simulink model "quad_copter_hybrid_vrft"  (R2016a)
settings: Solver=VariableStepAuto  StartTime=0.0  StopTime=10  RelTol=1e-3
undefined symbols (not defined in the file): DiscIntNeverNeededParam, HybridVRFTController, Mixer, PitchRateModel_dt, Ri_dt, Ts
settings Model: Creator=tibo  LastModifiedBy=tibo

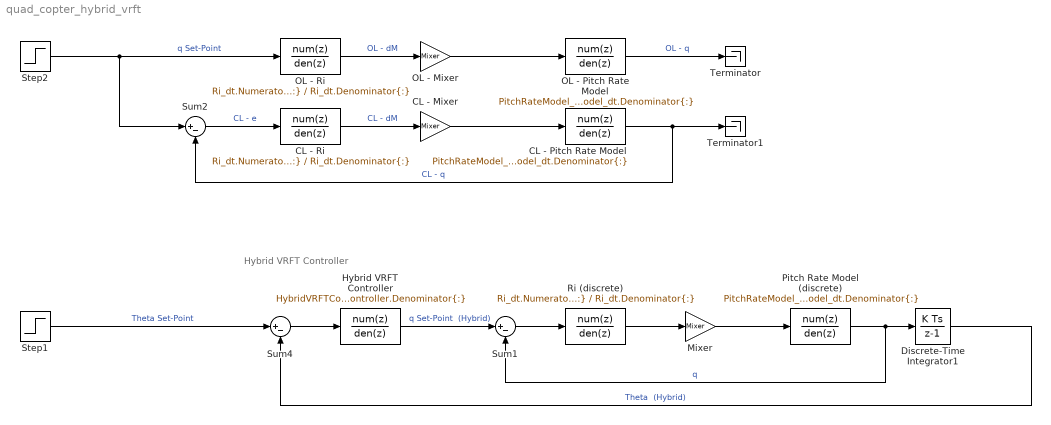
== system quad_copter_hybrid_vrft ==
  note: Hybrid VRFT Controller
  CL - Mixer : Gain  Gain=Mixer
  "CL - Pitch Rate Model " : DiscreteTransferFcn  Numerator=PitchRateModel_dt.Numerator{:}  Denominator=PitchRateModel_dt.Denominator{:}  SampleTime=Ts
  CL - Ri : DiscreteTransferFcn  Numerator=Ri_dt.Numerator{:}  Denominator=Ri_dt.Denominator{:}  SampleTime=Ts
  Discrete-Time Integrator1 : DiscreteIntegrator  InitialConditionSetting=State (most efficient)  SampleTime=Ts  ICPrevOutput=DiscIntNeverNeededParam  ICPrevScaledInput=DiscIntNeverNeededParam
  "Hybrid VRFT Controller " : DiscreteTransferFcn  Numerator=HybridVRFTController.Numerator{:}  Denominator=HybridVRFTController.Denominator{:}  SampleTime=Ts
  Mixer : Gain  Gain=Mixer
  OL - Mixer : Gain  Gain=Mixer
  "OL - Pitch Rate Model " : DiscreteTransferFcn  Numerator=PitchRateModel_dt.Numerator{:}  Denominator=PitchRateModel_dt.Denominator{:}  SampleTime=Ts
  OL - Ri : DiscreteTransferFcn  Numerator=Ri_dt.Numerator{:}  Denominator=Ri_dt.Denominator{:}  SampleTime=Ts
  Pitch Rate Model (discrete) : DiscreteTransferFcn  Numerator=PitchRateModel_dt.Numerator{:}  Denominator=PitchRateModel_dt.Denominator{:}  SampleTime=Ts
  Ri (discrete) : DiscreteTransferFcn  Numerator=Ri_dt.Numerator{:}  Denominator=Ri_dt.Denominator{:}  SampleTime=Ts
  Step1 : Step  After=.18  SampleTime=0
  Step2 : Step  Time=0  SampleTime=0
  Sum1 : Sum  Inputs=|+-
  Sum2 : Sum  Inputs=|+-
  Sum4 : Sum  Inputs=|+-
  Terminator : Terminator
  Terminator1 : Terminator
  wires:
  Step1/1 -> Sum4/1  "Theta Set-Point"
  Sum4/1 -> "Hybrid VRFT Controller "/1
  Discrete-Time Integrator1/1 -> Sum4/2  "Theta  (Hybrid)"
  "Hybrid VRFT Controller "/1 -> Sum1/1  "q Set-Point  (Hybrid)"
  Pitch Rate Model (discrete)/1 -> Sum1/2, Discrete-Time Integrator1/1  "q"
  Sum1/1 -> Ri (discrete)/1
  Ri (discrete)/1 -> Mixer/1
  Mixer/1 -> Pitch Rate Model (discrete)/1
  Step2/1 -> Sum2/1, OL - Ri/1  "q Set-Point"
  "OL - Pitch Rate Model "/1 -> Terminator/1  "OL - q"
  OL - Ri/1 -> OL - Mixer/1  "OL - dM"
  OL - Mixer/1 -> "OL - Pitch Rate Model "/1
  "CL - Pitch Rate Model "/1 -> Terminator1/1, Sum2/2  "CL - q"
  CL - Ri/1 -> CL - Mixer/1  "CL - dM"
  CL - Mixer/1 -> "CL - Pitch Rate Model "/1
  Sum2/1 -> CL - Ri/1  "CL - e"
